simulink model "prob1"  (R2020b)
settings: Solver=VariableStepAuto  StartTime=0.0  StopTime=10.0  RelTol=1e-3
model workspace (MAT data in the model file):
  b = Simulink.Parameter
  b.Value = 50
  b.DataType = 'auto'
  b.Dimensions = [1 1]
  k1 = Simulink.Parameter
  k1.Value = 50
  k1.DataType = 'auto'
  k1.Dimensions = [1 1]
  k2 = Simulink.Parameter
  k2.Value = 50
  k2.DataType = 'auto'
  k2.Dimensions = [1 1]
  m1 = Simulink.Parameter
  m1.Value = 100
  m1.DataType = 'auto'
  m1.Dimensions = [1 1]
  m2 = Simulink.Parameter
  m2.Value = 40
  m2.DataType = 'auto'
  m2.Dimensions = [1 1]
settings Model: Creator=Admin  LastModifiedBy=Admin

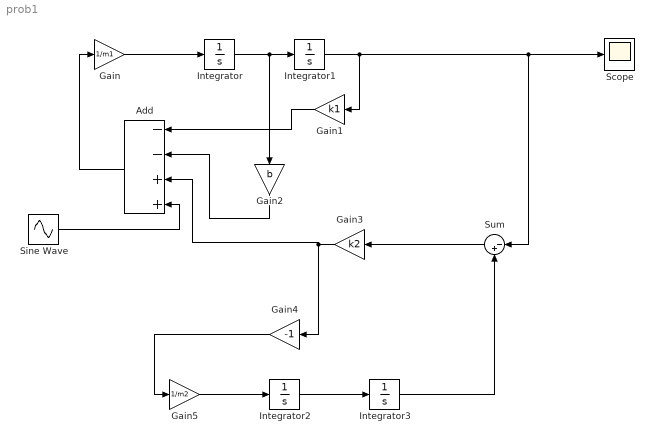
== system prob1 ==
  Add : Sum  Inputs=--++
  Gain : Gain  Gain=1/m1
  Gain1 : Gain  Gain=k1
  Gain2 : Gain  Gain=b
  Gain3 : Gain  Gain=k2
  Gain4 : Gain  Gain=-1
  Gain5 : Gain  Gain=1/m2
  Integrator{,1..3} (4 alike) : Integrator
  Scope : Scope
  Sine Wave : Sin  Amplitude=2  Frequency=10  SampleTime=0
  Sum : Sum  Inputs=|-+
  wires:
  Gain/1 -> Integrator/1
  Integrator/1 -> Gain2/1, Integrator1/1
  Integrator1/1 -> Scope/1, Sum/1, Gain1/1
  Gain1/1 -> Add/1
  Gain2/1 -> Add/2
  Gain3/1 -> Gain4/1, Add/3
  Sum/1 -> Gain3/1
  Gain4/1 -> Gain5/1
  Gain5/1 -> Integrator2/1
  Integrator2/1 -> Integrator3/1
  Integrator3/1 -> Sum/2
  Sine Wave/1 -> Add/4
  Add/1 -> Gain/1
